simulink model "Solar_Boost"  (R2022a)
settings: Solver=VariableStepAuto  StartTime=0.0  StopTime=1  RelTol=1e-3
libraries: spsSeriesRLCBranchLib x8, spsCurrentMeasurementLib x4, spsVoltageMeasurementLib x4, powerlib_extras x4, spsDiodeLib x2, spsIGBTDiodeLib x2, spsPVArrayLib x2, spsRMSLib x2, spspowerguiLib x2, spsPWMGeneratorDCDCLib x1
settings Model: Creator=nikke  LastModifiedBy=nikke

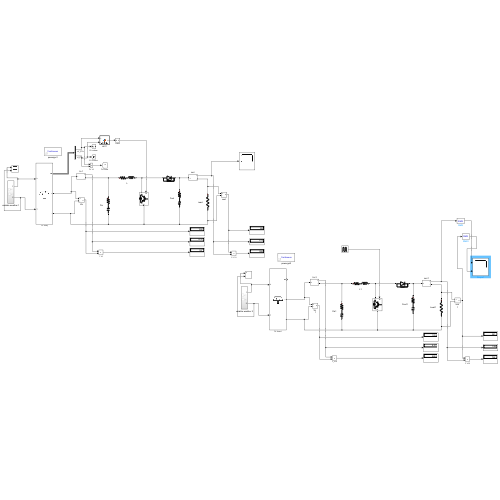
[thumbnail: Simulink's stored preview of the top-level diagram]
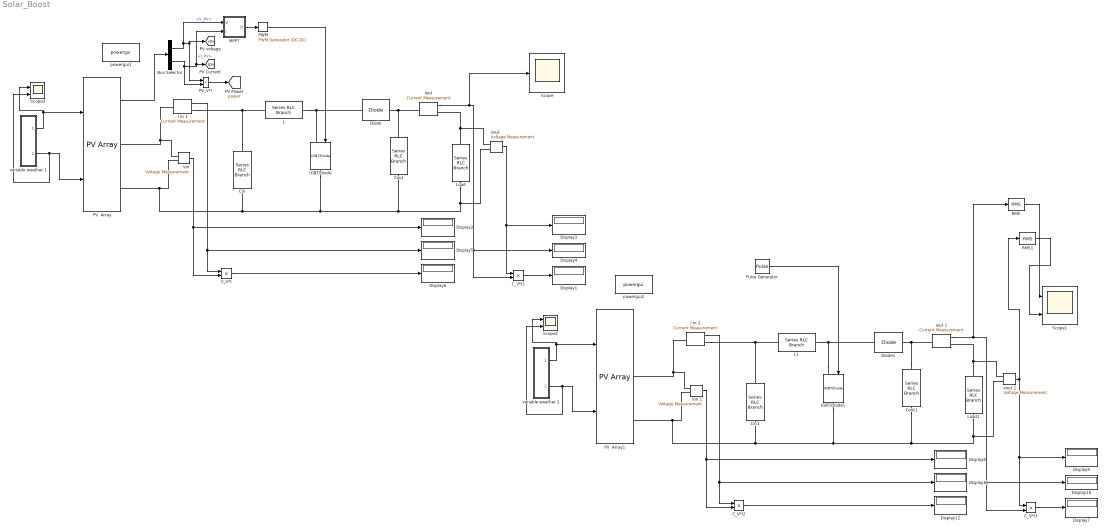
== system Solar_Boost ==
  Bus Selector : BusSelector  OutputSignals=V_PV,I_PV
  C_V*I{,1..3} (4 alike) : Product
  Cin : spsSeriesRLCBranchLib/Series RLC Branch  LConnTagsString=__new0  RConnTagsString=__new0  BranchType=RC  Resistance=1e-4  Inductance=1e-3  SetiL0=off  InitialCurrent=0  Capacitance=100e-6  Setx0=off  InitialVoltage=0  Measurements=None
  Cin1 : spsSeriesRLCBranchLib/Series RLC Branch  LConnTagsString=__new0  RConnTagsString=__new0  BranchType=RC  Resistance=1e-4  Inductance=1e-3  SetiL0=off  InitialCurrent=0  Capacitance=100e-6  Setx0=off  InitialVoltage=0  Measurements=None
  Cout : spsSeriesRLCBranchLib/Series RLC Branch  LConnTagsString=__new0  RConnTagsString=__new0  BranchType=RC  Resistance=0.0001  Inductance=1e-3  SetiL0=off  InitialCurrent=0  Capacitance=100e-6  Setx0=off  InitialVoltage=0  Measurements=None
  Cout1 : spsSeriesRLCBranchLib/Series RLC Branch  LConnTagsString=__new0  RConnTagsString=__new0  BranchType=RC  Resistance=0.0001  Inductance=1e-3  SetiL0=off  InitialCurrent=0  Capacitance=100e-6  Setx0=off  InitialVoltage=0  Measurements=None
  Diode : spsDiodeLib/Diode  Ron=0.001  Lon=0  Vf=0.8  IC=0  UseSnubber=off  Rs=500  Cs=250e-9  Measurements=off
  Diode1 : spsDiodeLib/Diode  Ron=0.001  Lon=0  Vf=0.8  IC=0  UseSnubber=off  Rs=500  Cs=250e-9  Measurements=off
  Display{1..12} (12 alike) : Display
  I in 1 : spsCurrentMeasurementLib/Current Measurement  PhasorSimulation=off  OutputType=Complex  PSBequivalent=0
  I in 2 : spsCurrentMeasurementLib/Current Measurement  PhasorSimulation=off  OutputType=Complex  PSBequivalent=0
  IGBT/Diode : spsIGBTDiodeLib/IGBT//Diode  Ron=1e-3  Rs=1e5  Cs=inf  Measurements=off
  IGBT/Diode1 : spsIGBTDiodeLib/IGBT//Diode  Ron=1e-3  Rs=1e5  Cs=inf  Measurements=off
  L : spsSeriesRLCBranchLib/Series RLC Branch  LConnTagsString=__new0  RConnTagsString=__new0  BranchType=RL  Resistance=0.1  Inductance=2e-3  SetiL0=off  InitialCurrent=0  Capacitance=100e-6  Setx0=off  InitialVoltage=0  Measurements=None
  L1 : spsSeriesRLCBranchLib/Series RLC Branch  LConnTagsString=__new0  RConnTagsString=__new0  BranchType=RL  Resistance=0.1  Inductance=2e-3  SetiL0=off  InitialCurrent=0  Capacitance=100e-6  Setx0=off  InitialVoltage=0  Measurements=None
  Load : spsSeriesRLCBranchLib/Series RLC Branch  LConnTagsString=__new0  RConnTagsString=__new0  BranchType=R  Resistance=200  Inductance=1e-3  SetiL0=off  InitialCurrent=0  Capacitance=100e-6  Setx0=off  InitialVoltage=0  Measurements=None
  Load1 : spsSeriesRLCBranchLib/Series RLC Branch  LConnTagsString=__new0  RConnTagsString=__new0  BranchType=R  Resistance=200  Inductance=1e-3  SetiL0=off  InitialCurrent=0  Capacitance=100e-6  Setx0=off  InitialVoltage=0  Measurements=None
  MPPT : MATLAB Function  TreatAsAtomicUnit=on
  PV  Array : spsPVArrayLib/PV Array  Npar=2  Nser=12  PlotType=array @ 1000 W/m2 & specified temperatures  S_vec="[ 1000  500  100 ]"  Temp_C_vec="[ 45 25  ]"  ModuleName=Tata Power Solar Systems TP140SBZ  PlotWhenSelected=off  Pm=139.6944  Ncell=36  Voc=22.25  Isc=8.66  Vm=17.44  Im=8.01  beta_Voc_pc=-0.33  alpha_Isc_pc=0.063799  beta_Voc=-0.073425  alpha_Isc=0.005525  IL=8.6872  I0=9.8965e-11  nI=0.95579  Rsh=88.7762  Rs=0.27837  RobustModel=off  RobustCellTemperature=313.3991  BAL=on  Tc=1e-6  Tfilter=5e-5
  PV  Array1 : spsPVArrayLib/PV Array  Npar=2  Nser=12  PlotType=array @ 1000 W/m2 & specified temperatures  S_vec="[ 1000  500  100 ]"  Temp_C_vec="[ 45 25  ]"  ModuleName=Tata Power Solar Systems TP140SBZ  PlotWhenSelected=off  Pm=139.6944  Ncell=36  Voc=22.25  Isc=8.66  Vm=17.44  Im=8.01  beta_Voc_pc=-0.33  alpha_Isc_pc=0.063799  beta_Voc=-0.073425  alpha_Isc=0.005525  IL=8.6872  I0=9.8965e-11  nI=0.95579  Rsh=88.7762  Rs=0.27837  RobustModel=off  RobustCellTemperature=313.3991  BAL=on  Tc=1e-6  Tfilter=5e-5
  PV_V*I : Product
  PWM : spsPWMGeneratorDCDCLib/PWM Generator (DC-DC)  Fsw=5000  Ts=5e-6
  Pulse Generator : DiscretePulseGenerator  PulseType=Time based  Period=1/1000  PulseWidth=50
  RMS : spsRMSLib/RMS  TrueRMS=on  Freq=50  RMSInit=120  Ts=0
  RMS1 : spsRMSLib/RMS  TrueRMS=on  Freq=50  RMSInit=120  Ts=0
  Scope : Scope
  Scope1 : Scope  NumInputPorts=2
  Scope2 : Scope  NumInputPorts=2
  Scope3 : Scope  NumInputPorts=2
  "Vin " : spsVoltageMeasurementLib/Voltage Measurement  PhasorSimulation=off  OutputType=Complex  PSBequivalent=0
  Vin 1 : spsVoltageMeasurementLib/Voltage Measurement  PhasorSimulation=off  OutputType=Complex  PSBequivalent=0
  "iout " : spsCurrentMeasurementLib/Current Measurement  PhasorSimulation=off  OutputType=Complex  PSBequivalent=0
  iout 1 : spsCurrentMeasurementLib/Current Measurement  PhasorSimulation=off  OutputType=Complex  PSBequivalent=0
  powergui1 : spspowerguiLib/powergui  Priority=1  SimulationMode=Continuous  SampleTime=50e-6  frequency=60  Iterations=50  frequencyindice=0  Pbase=100e6  ErrMax=1e-4  UnitsV=kV  UnitsW=MW  buscounter=0  FunctionMessages=off  echomessages=off  EnableUseOfTLC=off  CurrentSourceSwitches=off  DisableSnubberDevices=off  DisableRonSwitches=off  DisableVfSwitches=off  DisplayEquations=off  AutomaticDiscreteSolvers=off  SolverType=Tustin/Backward Euler (TBE)  Interpol=off  ExternalGateDelay=off  methode=off  Ts=100  x0status=blocks  SPID=on  SwTol=0  HookPort=off  NonlinearTolerance=1e-4  nMaxIteration=100  ContinueOnMaxIteration=off  RestoreLinks=warning  ResistiveCurrentMeasurement=off  Frange=[0:2:500]  Ylog=off  Xlog=on  ShowGrid=off  save=off  variable=ZData  structure=0  ZoomFFT=off  StartTime=0.0  cycles=1  DisplayStyle=1  fundamental=60  FreqAxis=off  MaxFrequency=1000  frequencyindicesteady=1  RmsSteady=1  display=off
  powergui2 : spspowerguiLib/powergui  Priority=1  SimulationMode=Continuous  SampleTime=50e-6  frequency=60  Iterations=50  frequencyindice=0  Pbase=100e6  ErrMax=1e-4  UnitsV=kV  UnitsW=MW  buscounter=0  FunctionMessages=off  echomessages=off  EnableUseOfTLC=off  CurrentSourceSwitches=off  DisableSnubberDevices=off  DisableRonSwitches=off  DisableVfSwitches=off  DisplayEquations=off  AutomaticDiscreteSolvers=off  SolverType=Tustin/Backward Euler (TBE)  Interpol=off  ExternalGateDelay=off  methode=off  Ts=100  x0status=blocks  SPID=on  SwTol=0  HookPort=off  NonlinearTolerance=1e-4  nMaxIteration=100  ContinueOnMaxIteration=off  RestoreLinks=warning  ResistiveCurrentMeasurement=off  Frange=[0:2:500]  Ylog=off  Xlog=on  ShowGrid=off  save=off  variable=ZData  structure=0  ZoomFFT=off  StartTime=0.0  cycles=1  DisplayStyle=1  fundamental=60  FreqAxis=off  MaxFrequency=1000  frequencyindicesteady=1  RmsSteady=1  display=off
  variable weather 1 : Subsystem
  variable weather 2 : Subsystem
  "vout " : spsVoltageMeasurementLib/Voltage Measurement  PhasorSimulation=off  OutputType=Complex  PSBequivalent=0
  vout 1 : spsVoltageMeasurementLib/Voltage Measurement  PhasorSimulation=off  OutputType=Complex  PSBequivalent=0
  tag scope: ipv=global, power=global, vpv=global
  wires:
  "vout "/1 -> Display3/1, C_V*I1/1
  C_V*I1/1 -> Display1/1
  C_V*I/1 -> Display6/1
  I in 1/1 -> Display5/1, C_V*I/1
  "Vin "/1 -> C_V*I/2, Display2/1
  "iout "/1 -> Scope/1, Display4/1, C_V*I1/2
  PWM/1 -> IGBT/Diode/1
  MPPT/1(D) -> PWM/1
  Bus Selector/1 -> [vpv], PV_V*I/1, MPPT/1(V)  "<V_PV>"
  Bus Selector/2 -> MPPT/2(I), [ipv], PV_V*I/2  "<I_PV>"
  PV_V*I/1 -> [power]
  PV  Array/1 -> Bus Selector/1
  variable weather 1/2(Out2) -> PV  Array/2, Scope3/2
  variable weather 1/1(Out1) -> PV  Array/1, Scope3/1
  variable weather 2/1(Out1) -> PV  Array1/1, Scope2/1
  iout 1/1 -> RMS/1, Display10/1, C_V*I3/2
  variable weather 2/2(Out2) -> PV  Array1/2, Scope2/2
  Vin 1/1 -> C_V*I2/2, Display8/1
  vout 1/1 -> Display9/1, C_V*I3/1, RMS1/1
  C_V*I3/1 -> Display7/1
  C_V*I2/1 -> Display12/1
  I in 2/1 -> Display11/1, C_V*I2/1
  Pulse Generator/1 -> IGBT/Diode1/1
  RMS/1 -> Scope1/1
  RMS1/1 -> Scope1/2
  connections:
  Load/RConn1 -- Cout/RConn1 -- "Vin "/LConn2 -- PV  Array/RConn2 -- Cin/RConn1 -- IGBT/Diode/RConn1 -- "vout "/LConn2
  I in 1/LConn1 -- PV  Array/RConn1 -- "Vin "/LConn1
  Cin/LConn1 -- L/LConn1 -- I in 1/RConn1
  L/RConn1 -- Diode/LConn1 -- IGBT/Diode/LConn1
  Diode/RConn1 -- "iout "/LConn1 -- Cout/LConn1
  Load/LConn1 -- "vout "/LConn1 -- "iout "/RConn1
  PV  Array1/RConn2 -- Load1/RConn1 -- vout 1/LConn2 -- Cout1/RConn1 -- IGBT/Diode1/RConn1 -- Cin1/RConn1 -- Vin 1/LConn2
  IGBT/Diode1/LConn1 -- L1/RConn1 -- Diode1/LConn1
  I in 2/RConn1 -- Cin1/LConn1 -- L1/LConn1
  iout 1/RConn1 -- Load1/LConn1 -- vout 1/LConn1
  Cout1/LConn1 -- Diode1/RConn1 -- iout 1/LConn1
  Vin 1/LConn1 -- I in 2/LConn1 -- PV  Array1/RConn1

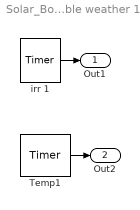
== system Solar_Boost/variable weather 1 ==
  Temp1 : powerlib_extras/Control  Blocks/Timer  t=[0 .1 .2 .3 .4 .5 .6 .7 .8 .9 1 ]  e=[20 23 25 25 26 27 28 25 25 25 25]
      settings: SourceProductBaseCode=PS
  irr 1 : powerlib_extras/Control  Blocks/Timer  t=[0 0.05 0.1 .15 .2 .25 .3 .35 0.4 .45 .5 ]  e=[250 500 500 500 600 700 800 1000 1000 700 500 ]
      settings: SourceProductBaseCode=PS
  Out1 : Outport
  Out2 : Outport  Port=2
  wires:
  irr 1/1 -> Out1/1
  Temp1/1 -> Out2/1

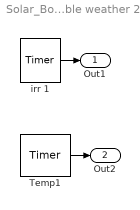
== system Solar_Boost/variable weather 2 ==
  Temp1 : powerlib_extras/Control  Blocks/Timer  t=[0 .1 .2 .3 .4 .5 .6 .7 .8 .9 1 ]  e=[20 23 25 25 26 27 28 25 25 25 25]
      settings: SourceProductBaseCode=PS
  irr 1 : powerlib_extras/Control  Blocks/Timer  t=[0 0.05 0.1 .15 .2 .25 .3 .35 0.4 .45 .5 ]  e=[250 500 500 500 600 700 800 1000 1000 700 500 ]
      settings: SourceProductBaseCode=PS
  Out1 : Outport
  Out2 : Outport  Port=2
  wires:
  irr 1/1 -> Out1/1
  Temp1/1 -> Out2/1

== matlab function Solar_Boost/MPPT ==
  settings: updateMethod=DISCRETE
  data: V input; D output; I input
% author : Saad MOTAHHIR
% f=1000hz
function D  = ModINC(V, I)


Dinit = 0.6;  %Initial value for D output
Dmax = 0.65;   %Maximum value for D
Dmin = 0.1;   %Minimum value for D
deltaD = 0.0007; %Increment value used to increase/decrease the duty cycle D

  
persistent Vold Pold Dold Iold M;

dataType = 'double';

if isempty(Vold)
    Vold=0;
    Pold=0;
    Iold=0;
    Dold=Dinit;
    M=1;
end
P= V*I;
dV= V - Vold;
dP= P - Pold;
dI= I - Iold;
M=abs(dP);

if M < 0.005
    D=Dold;
else
    if dV == 0
        if dI == 0
            D=Dold;
        elseif dI>0
            D=Dold - (M*deltaD);
        else 
            D=Dold + (M*deltaD);
        end    
    else
        if dI/dV == -I/V
            D=Dold;
        elseif dI/dV>-I/V    
           D=Dold - (M*deltaD);
        else
           D=Dold + (M*deltaD);  
        end  
    end    
end

if D >= Dmax | D<= Dmin
    D=Dold;
end

Dold=D;
Vold=V;
Pold=P;
Iold=I;
